simulink model "MSabc_TPM1Base0x2830x291"  (R2023b)
settings: Solver=ode45  StartTime=0.0  StopTime=0.5  MaxStep=h/10  RelTol=1e-3  EnableMultiTasking=on
model workspace (MAT data in the model file):
  J = 0.004
  Lc_v = 0.00255
  R_v = 0.13
  Vmax = 530
  fv = 0.08
  p = 4
  psid0_v = 0.222
values from neighbouring files (symbols this model uses):
  h = 50e-6    (= 5e-05)    [MotorDat_MSTPM1 (1).m]    (also in ParamMinduction0.m; parametres.m = 1e-05)
libraries: simulink x1, spsThreePhaseSineGeneratorLib x1
settings Model: Creator=dgrenier  LastModifiedBy=boris
settings SolverCC: AlgebraicLoopSolver=TrustRegion
settings DataIOCC: LimitDataPoints=on  SaveFormat=Array  SignalLoggingSaveFormat=ModelDataLogs  ReturnWorkspaceOutputs=off
settings OptimizationCC: ExpressionDepthLimit=2147483647  InitFltsAndDblsToZero=on  LifeSpan=inf
settings DebuggingCC: SaveWithParameterizedLinksMsg=none  UnderspecifiedInitializationDetection=Classic  MergeDetectMultiDrivingBlocksExec=none  SignalResolutionControl=TryResolveAllWithWarning  SolverPrmCheckMsg=warning  MultiTaskDSMMsg=warning  MultiTaskCondExecSysMsg=none  FcnCallInpInsideContextMsg=warning  UnconnectedInputMsg=warning  UnconnectedOutputMsg=warning  UnconnectedLineMsg=warning  StateNameClashWarn=warning  SFUnexpectedBacktrackingDiag=warning  SFNoUnconditionalDefaultTransitionDiag=warning  SFExecutionAtInitializationDiag=none  ArithmeticOperatorsInVariantConditions=warning
settings HardwareCC: ProdBitPerPointer=32  ProdBitPerSizeT=32  ProdBitPerPtrDiffT=32  ProdLargestAtomicFloat=None  ProdIntDivRoundTo=Undefined  ProdEndianess=Unspecified  ProdWordSize=32  ProdHWDeviceType=32-bit Generic
settings ModelReferenceCC: EnableRefExpFcnMdlSchedulingChecks=on  PropagateSignalLabelsOutOfModel=off
settings SFSimCC: SimUseLocalCustomCode=off  CustomCodeUndefinedFunction=UseInterfaceOnly
settings RTWCC: RTWUseLocalCustomCode=off  DLArmComputeVersion=19.05
settings CodeAppCC: StateflowObjectComments=on
settings GRTTargetCC: TargetFcnLib=ansi_tfl_tmw.mat  TargetLangStandard=C89/C90 (ANSI)  CombineOutputUpdateFcns=off  GRTInterface=on
settings ConfigComp: CovMetricSettings=dw  CovSaveCumulativeToWorkspaceVar=on  CovSaveSingleToWorkspaceVar=on  CovExternalEMLEnable=off  CovSFcnEnable=off

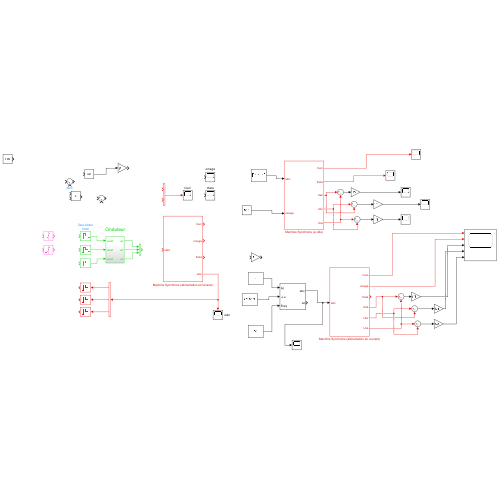
[thumbnail: Simulink's stored preview of the top-level diagram]
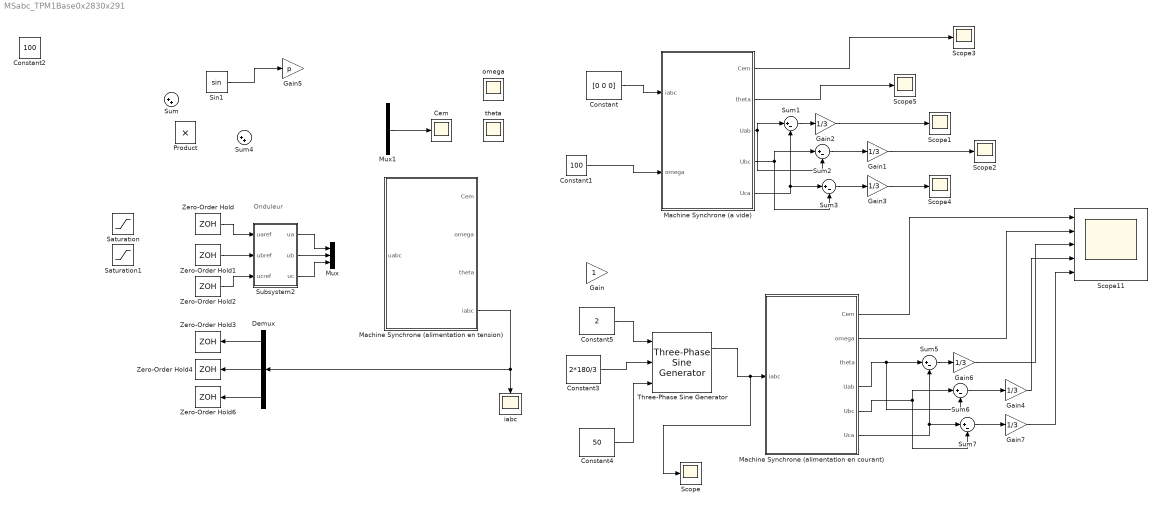
== system MSabc_TPM1Base0x2830x291 ==
  note: Onduleur
  Cem : Scope
  Constant : Constant  Value=[0 0 0]
  Constant1 : Constant  Value=100
  Constant2 : Constant  Value=100
  Constant3 : Constant  Value=2*180/3
  Constant4 : Constant  Value=50
  Constant5 : Constant  Value=2
  Demux : Demux  Outputs=3
  Gain : Gain
  Gain{1..4,6..7} (6 alike) : Gain  Gain=1/3
  Gain5 : Gain  Gain=p
  Machine Synchrone (a vide) : Subsystem
  Machine Synchrone (alimentation en courant) : Subsystem
  Machine Synchrone (alimentation en tension) : Subsystem
  Mux : Mux  Inputs=3
  Mux1 : Mux  Inputs=2
  Product : Product
  Saturation : Saturate  UpperLimit=Vmax/2  LowerLimit=-Vmax/2
  Saturation1 : Saturate  UpperLimit=Vmax/2  LowerLimit=-Vmax/2
  Scope{,1..5} (6 alike) : Scope
  Scope11 : Scope  NumInputPorts=5
  Sin1 : Trigonometry
  Subsystem2 : Subsystem
  Sum : Sum  Inputs=|++
  Sum{1..3,5..7} (6 alike) : Sum  Inputs=|+-
  Sum4 : Sum  Inputs=|++
  Three-Phase Sine Generator : spsThreePhaseSineGeneratorLib/Three-Phase Sine Generator  Ts=0
      settings: LibrarySourceBlock=|
      | sps_lib/Sources/Signal Generator Sources/Three-Phase
      | Sine Generator
  Zero-Order Hold{,1..4,6} (6 alike) : ZeroOrderHold  SampleTime=h
  iabc : Scope
  omega : Scope
  theta : Scope
  wires:
  Subsystem2/1(ua) -> Mux/1
  Subsystem2/2(ub) -> Mux/2
  Subsystem2/3(uc) -> Mux/3
  Mux1/1 -> Cem/1
  Zero-Order Hold/1 -> Subsystem2/1(uaref)
  Zero-Order Hold1/1 -> Subsystem2/2(ubref)
  Zero-Order Hold2/1 -> Subsystem2/3(ucref)
  Demux/1 -> Zero-Order Hold3/1
  Demux/2 -> Zero-Order Hold4/1
  Demux/3 -> Zero-Order Hold6/1
  Machine Synchrone (alimentation en tension)/4(iabc) -> Demux/1, iabc/1
  Constant/1 -> Machine Synchrone (a vide)/1(iabc)
  Constant1/1 -> Machine Synchrone (a vide)/2(omega)
  Sin1/1 -> Gain5/1
  Machine Synchrone (a vide)/3(Uab) -> Sum1/1, Sum2/2
  Machine Synchrone (a vide)/5(Uca) -> Sum3/1, Sum1/2
  Sum1/1 -> Gain2/1
  Gain2/1 -> Scope1/1
  Sum2/1 -> Gain1/1
  Machine Synchrone (a vide)/4(Ubc) -> Sum2/1, Sum3/2
  Gain1/1 -> Scope2/1
  Sum3/1 -> Gain3/1
  Gain3/1 -> Scope4/1
  Machine Synchrone (a vide)/1(Cem) -> Scope3/1
  Machine Synchrone (a vide)/2(theta) -> Scope5/1
  Three-Phase Sine Generator/1 -> Scope/1, Machine Synchrone (alimentation en courant)/1(iabc)
  Constant3/1 -> Three-Phase Sine Generator/2
  Sum6/1 -> Gain4/1
  Sum7/1 -> Gain7/1
  Sum5/1 -> Gain6/1
  Machine Synchrone (alimentation en courant)/5(Ubc) -> Sum6/1, Sum7/2
  Machine Synchrone (alimentation en courant)/6(Uca) -> Sum7/1, Sum5/2
  Gain4/1 -> Scope11/4
  Gain6/1 -> Scope11/3
  Gain7/1 -> Scope11/5
  Machine Synchrone (alimentation en courant)/4(Uab) -> Sum5/1, Sum6/2
  Machine Synchrone (alimentation en courant)/1(Cem) -> Scope11/1
  Machine Synchrone (alimentation en courant)/2(omega) -> Scope11/2
  Constant4/1 -> Three-Phase Sine Generator/3
  Constant5/1 -> Three-Phase Sine Generator/1

== system MSabc_TPM1Base0x2830x291/Machine Synchrone (a vide) ==
  iabc : Inport
  omega : Inport  Port=2
  Integrator1 : Integrator  InitialCondition=pi/6  WrapState=on
  Machine Synchrone1 : Subsystem
  Sum : Sum  Inputs=|+-
  Sum1 : Sum  Inputs=|+-
  Sum2 : Sum  Inputs=-+|
  Cem : Outport
  theta : Outport  Port=2
  Uab : Outport  Port=3
  Ubc : Outport  Port=4
  Uca : Outport  Port=5
  wires:
  iabc/1 -> Machine Synchrone1/3(iabc)
  Integrator1/1 -> Machine Synchrone1/2(thetam), theta/1
  Machine Synchrone1/1(Cem) -> Cem/1
  omega/1 -> Machine Synchrone1/1(omegam), Integrator1/1
  Machine Synchrone1/2(ua) -> Sum2/1, Sum/1
  Machine Synchrone1/3(ub) -> Sum/2, Sum1/1
  Sum1/1 -> Ubc/1
  Sum/1 -> Uab/1
  Machine Synchrone1/4(uc) -> Sum1/2, Sum2/2
  Sum2/1 -> Uca/1

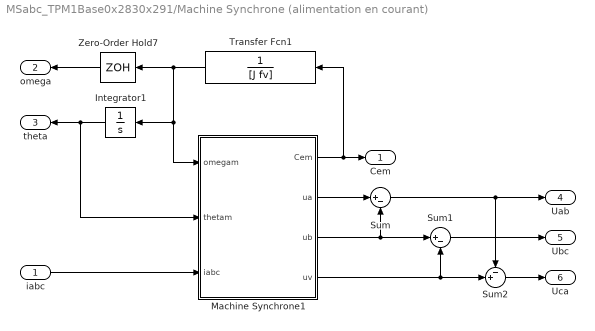
== system MSabc_TPM1Base0x2830x291/Machine Synchrone (alimentation en courant) ==
  iabc : Inport
  Integrator1 : Integrator  InitialCondition=pi/6  WrapState=on
  Machine Synchrone1 : Subsystem
  Sum : Sum  Inputs=|+-
  Sum1 : Sum  Inputs=|+-
  Sum2 : Sum  Inputs=-+|
  Transfer Fcn1 : TransferFcn  Denominator=[J fv]
  Zero-Order Hold7 : ZeroOrderHold  SampleTime=h
  Cem : Outport
  omega : Outport  Port=2
  theta : Outport  Port=3
  Uab : Outport  Port=4
  Ubc : Outport  Port=5
  Uca : Outport  Port=6
  wires:
  iabc/1 -> Machine Synchrone1/3(iabc)
  Integrator1/1 -> Machine Synchrone1/2(thetam), theta/1
  Transfer Fcn1/1 -> Machine Synchrone1/1(omegam), Integrator1/1, Zero-Order Hold7/1
  Zero-Order Hold7/1 -> omega/1
  Machine Synchrone1/1(Cem) -> Cem/1, Transfer Fcn1/1
  Sum/1 -> Sum2/1, Uab/1
  Machine Synchrone1/4(uv) -> Sum2/2, Sum1/2
  Machine Synchrone1/3(ub) -> Sum/2, Sum1/1
  Sum1/1 -> Ubc/1
  Sum2/1 -> Uca/1
  Machine Synchrone1/2(ua) -> Sum/1

== system MSabc_TPM1Base0x2830x291/Machine Synchrone (alimentation en tension) ==
  uabc : Inport
  Integrator : Integrator  InitialCondition=pi/6  WrapState=on
  Machine Synchrone : Subsystem
  Transfer Fcn4 : TransferFcn  Denominator=[J fv]
  Zero-Order Hold5 : ZeroOrderHold  SampleTime=h
  Cem : Outport
  omega : Outport  Port=2
  theta : Outport  Port=3
  iabc : Outport  Port=4
  wires:
  Zero-Order Hold5/1 -> omega/1
  Machine Synchrone/2(iabc) -> iabc/1
  Integrator/1 -> Machine Synchrone/2(thetam), theta/1
  uabc/1 -> Machine Synchrone/3(uabc)
  Machine Synchrone/1(Cem) -> Cem/1, Transfer Fcn4/1
  Transfer Fcn4/1 -> Machine Synchrone/1(omegam), Integrator/1, Zero-Order Hold5/1

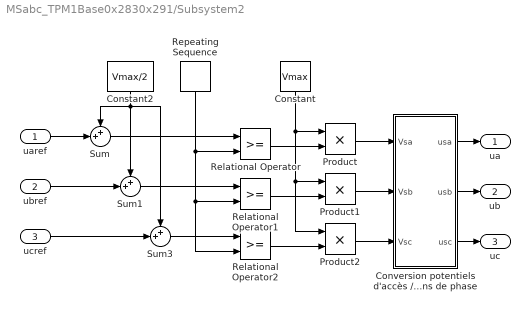
== system MSabc_TPM1Base0x2830x291/Subsystem2 ==
  uaref : Inport
  ubref : Inport  Port=2
  ucref : Inport  Port=3
  Constant : Constant  Value=Vmax
  Constant2 : Constant  Value=Vmax/2
  Conversion potentiels d'accès / tensions de phase : Subsystem
  Product : Product  RndMeth=Zero
  Product1 : Product  RndMeth=Zero
  Product2 : Product  RndMeth=Zero
  Relational Operator : RelationalOperator  OutDataTypeStr=boolean  ZeroCross=off  InputSameDT=off
  Relational Operator1 : RelationalOperator  OutDataTypeStr=boolean  ZeroCross=off  InputSameDT=off
  Relational Operator2 : RelationalOperator  OutDataTypeStr=boolean  ZeroCross=off  InputSameDT=off
  Repeating Sequence : simulink/Sources/Repeating Sequence  rep_seq_t=[0 h 2*h]  rep_seq_y=[0 Vmax 0]
  Sum : Sum  Inputs=++|
  Sum1 : Sum  Inputs=++|
  Sum3 : Sum  Inputs=++|
  ua : Outport
  ub : Outport  Port=2
  uc : Outport  Port=3
  wires:
  Constant2/1 -> Sum3/1, Sum/1, Sum1/1
  Product2/1 -> Conversion potentiels d'accès / tensions de phase/3(Vsc)
  Product1/1 -> Conversion potentiels d'accès / tensions de phase/2(Vsb)
  Product/1 -> Conversion potentiels d'accès / tensions de phase/1(Vsa)
  Relational Operator2/1 -> Product2/2
  Sum3/1 -> Relational Operator2/1
  Sum1/1 -> Relational Operator1/1
  Sum/1 -> Relational Operator/1
  Relational Operator1/1 -> Product1/2
  Constant/1 -> Product2/1, Product1/1, Product/1
  Relational Operator/1 -> Product/2
  Repeating Sequence/1 -> Relational Operator2/2, Relational Operator1/2, Relational Operator/2
  Conversion potentiels d'accès / tensions de phase/3(usc) -> uc/1
  Conversion potentiels d'accès / tensions de phase/2(usb) -> ub/1
  Conversion potentiels d'accès / tensions de phase/1(usa) -> ua/1
  ucref/1 -> Sum3/2
  uaref/1 -> Sum/2
  ubref/1 -> Sum1/2

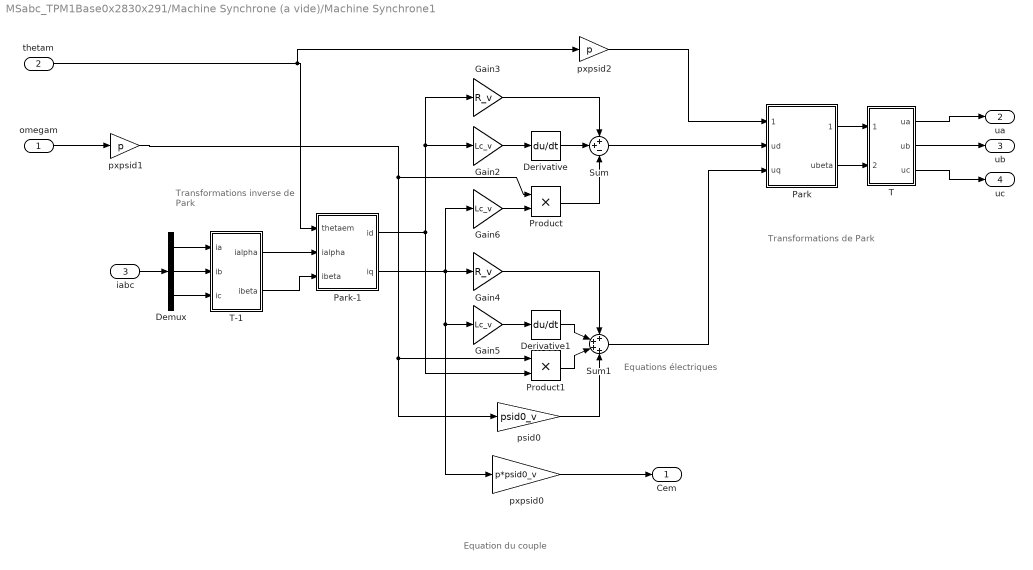
== system MSabc_TPM1Base0x2830x291/Machine Synchrone (a vide)/Machine Synchrone1 ==
  note: Transformations de Park
  note: Transformations
      | inverse de Park
  note: Equation du couple
  note: Equations électriques
  omegam : Inport
  thetam : Inport  Port=2
  iabc : Inport  Port=3
  Demux : Demux  Outputs=3
  Derivative : Derivative
  Derivative1 : Derivative
  Gain2 : Gain  Gain=Lc_v
  Gain3 : Gain  Gain=R_v
  Gain4 : Gain  Gain=R_v
  Gain5 : Gain  Gain=Lc_v
  Gain6 : Gain  Gain=Lc_v
  Park : Subsystem
  Park-1 : Subsystem
  Product : Product  RndMeth=Zero
  Product1 : Product  RndMeth=Zero
  Sum : Sum  Inputs=++-
  Sum1 : Sum  Inputs=++++
  T : Subsystem
  T-1 : Subsystem
  psid0 : Gain  Gain=psid0_v
  pxpsid0 : Gain  Gain=p*psid0_v
  pxpsid1 : Gain  Gain=p
  pxpsid2 : Gain  Gain=p
  Cem : Outport
  ua : Outport  Port=2
  ub : Outport  Port=3
  uc : Outport  Port=4
  wires:
  pxpsid0/1 -> Cem/1
  T/3(uc) -> uc/1
  T/2(ub) -> ub/1
  Demux/3 -> T-1/3(ic)
  Demux/2 -> T-1/2(ib)
  Park/1(ualpha) -> T/1(ialpha)
  Park/2(ubeta) -> T/2(ibeta)
  Sum/1 -> Park/2(ud)
  pxpsid1/1 -> psid0/1, Product1/1, Product/1
  T-1/2(ibeta) -> Park-1/3(ibeta)
  T-1/1(ialpha) -> Park-1/2(ialpha)
  T/1(ua) -> ua/1
  iabc/1 -> Demux/1
  Demux/1 -> T-1/1(ia)
  omegam/1 -> pxpsid1/1
  thetam/1 -> pxpsid2/1, Park-1/1(thetaem)
  Park-1/1(id) -> Product1/2, Gain3/1, Gain2/1
  Gain2/1 -> Derivative/1
  Gain3/1 -> Sum/1
  Derivative/1 -> Sum/2
  Product/1 -> Sum/3
  Gain6/1 -> Product/2
  Park-1/2(iq) -> Gain5/1, pxpsid0/1, Gain4/1, Gain6/1
  Gain5/1 -> Derivative1/1
  Derivative1/1 -> Sum1/2
  Gain4/1 -> Sum1/1
  Product1/1 -> Sum1/3
  psid0/1 -> Sum1/4
  Sum1/1 -> Park/3(uq)
  pxpsid2/1 -> Park/1(thetaem)

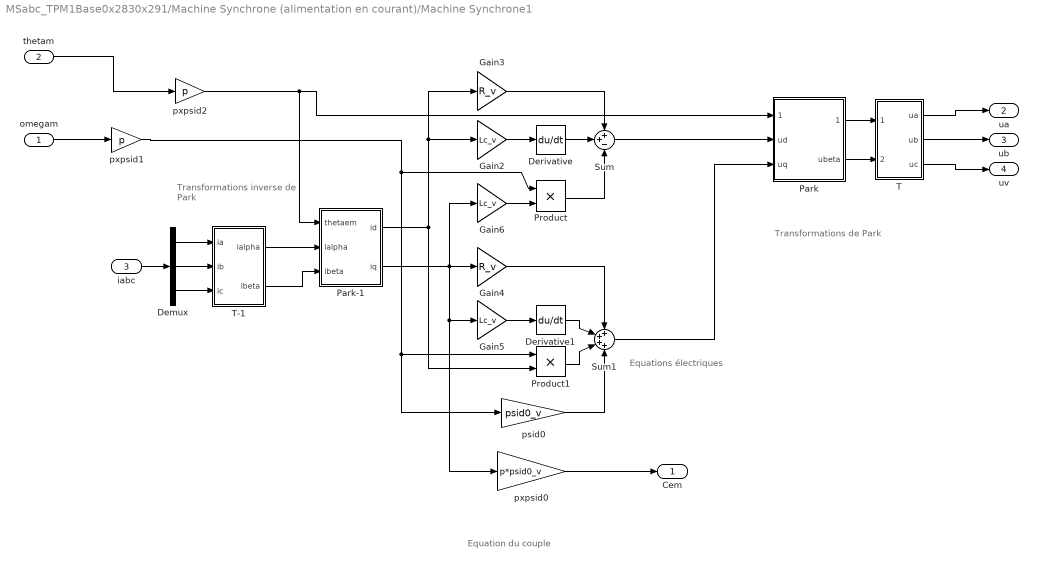
== system MSabc_TPM1Base0x2830x291/Machine Synchrone (alimentation en courant)/Machine Synchrone1 ==
  note: Transformations de Park
  note: Transformations
      | inverse de Park
  note: Equation du couple
  note: Equations électriques
  omegam : Inport
  thetam : Inport  Port=2
  iabc : Inport  Port=3
  Demux : Demux  Outputs=3
  Derivative : Derivative
  Derivative1 : Derivative
  Gain2 : Gain  Gain=Lc_v
  Gain3 : Gain  Gain=R_v
  Gain4 : Gain  Gain=R_v
  Gain5 : Gain  Gain=Lc_v
  Gain6 : Gain  Gain=Lc_v
  Park : Subsystem
  Park-1 : Subsystem
  Product : Product  RndMeth=Zero
  Product1 : Product  RndMeth=Zero
  Sum : Sum  Inputs=++-
  Sum1 : Sum  Inputs=++++
  T : Subsystem
  T-1 : Subsystem
  psid0 : Gain  Gain=psid0_v
  pxpsid0 : Gain  Gain=p*psid0_v
  pxpsid1 : Gain  Gain=p
  pxpsid2 : Gain  Gain=p
  Cem : Outport
  ua : Outport  Port=2
  ub : Outport  Port=3
  uv : Outport  Port=4
  wires:
  pxpsid0/1 -> Cem/1
  T/2(ub) -> ub/1
  Demux/3 -> T-1/3(ic)
  Demux/2 -> T-1/2(ib)
  Park/1(ualpha) -> T/1(ialpha)
  Park/2(ubeta) -> T/2(ibeta)
  Sum/1 -> Park/2(ud)
  pxpsid1/1 -> psid0/1, Product1/1, Product/1
  T-1/2(ibeta) -> Park-1/3(ibeta)
  T-1/1(ialpha) -> Park-1/2(ialpha)
  T/1(ua) -> ua/1
  iabc/1 -> Demux/1
  Demux/1 -> T-1/1(ia)
  omegam/1 -> pxpsid1/1
  Park-1/1(id) -> Product1/2, Gain3/1, Gain2/1
  Gain2/1 -> Derivative/1
  Gain3/1 -> Sum/1
  Derivative/1 -> Sum/2
  Product/1 -> Sum/3
  Gain6/1 -> Product/2
  Park-1/2(iq) -> Gain5/1, pxpsid0/1, Gain4/1, Gain6/1
  Gain5/1 -> Derivative1/1
  Derivative1/1 -> Sum1/2
  Gain4/1 -> Sum1/1
  Product1/1 -> Sum1/3
  psid0/1 -> Sum1/4
  Sum1/1 -> Park/3(uq)
  T/3(uc) -> uv/1
  pxpsid2/1 -> Park-1/1(thetaem), Park/1(thetaem)
  thetam/1 -> pxpsid2/1

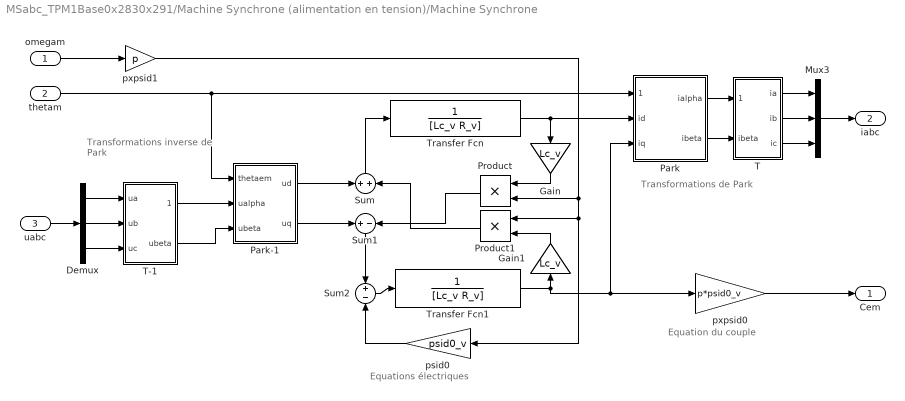
== system MSabc_TPM1Base0x2830x291/Machine Synchrone (alimentation en tension)/Machine Synchrone ==
  note: Transformations de Park
  note: Transformations
      | inverse de Park
  note: Equation du couple
  note: Equations électriques
  omegam : Inport
  thetam : Inport  Port=2
  uabc : Inport  Port=3
  Demux : Demux  Outputs=3
  Gain : Gain  Gain=Lc_v
  Gain1 : Gain  Gain=Lc_v
  Mux3 : Mux  Inputs=3
  Park : Subsystem
  Park-1 : Subsystem
  Product : Product  RndMeth=Zero
  Product1 : Product  RndMeth=Zero
  Sum : Sum  Inputs=+|+
  Sum1 : Sum  Inputs=+|-
  Sum2 : Sum  Inputs=+|-
  T : Subsystem
  T-1 : Subsystem
  Transfer Fcn : TransferFcn  Denominator=[Lc_v R_v]
  Transfer Fcn1 : TransferFcn  Denominator=[Lc_v R_v]
  psid0 : Gain  Gain=psid0_v
  pxpsid0 : Gain  Gain=p*psid0_v
  pxpsid1 : Gain  Gain=p
  Cem : Outport
  iabc : Outport  Port=2
  wires:
  pxpsid0/1 -> Cem/1
  T/3(ic) -> Mux3/3
  T/2(ib) -> Mux3/2
  Demux/3 -> T-1/3(uc)
  Demux/2 -> T-1/2(ub)
  Park/1(ialpha) -> T/1(ialpha)
  Park/2(ibeta) -> T/2(ibeta)
  psid0/1 -> Sum2/2
  Gain1/1 -> Product1/2
  Transfer Fcn1/1 -> pxpsid0/1, Park/3(iq), Gain1/1
  Sum2/1 -> Transfer Fcn1/1
  Sum1/1 -> Sum2/1
  Sum/1 -> Transfer Fcn/1
  Product1/1 -> Sum/2
  Product/1 -> Sum1/2
  Transfer Fcn/1 -> Gain/1, Park/2(id)
  Gain/1 -> Product/1
  Park-1/2(uq) -> Sum1/1
  Park-1/1(ud) -> Sum/1
  T-1/2(ubeta) -> Park-1/3(ubeta)
  T-1/1(ualpha) -> Park-1/2(ualpha)
  T/1(ia) -> Mux3/1
  Mux3/1 -> iabc/1
  uabc/1 -> Demux/1
  Demux/1 -> T-1/1(ua)
  omegam/1 -> pxpsid1/1
  pxpsid1/1 -> Product/2, Product1/1, psid0/1
  thetam/1 -> Park/1(thetaem), Park-1/1(thetaem)

== system MSabc_TPM1Base0x2830x291/Subsystem2/Conversion potentiels d'accès // tensions de phase ==
  Vsa : Inport
  Vsb : Inport  Port=2
  Vsc : Inport  Port=3
  Gain : Gain  Gain=1/3
  Sum : Sum  Inputs=+++
  Sum1 : Sum  Inputs=-+|
  Sum2 : Sum  Inputs=-+|
  Sum3 : Sum  Inputs=-+|
  usa : Outport
  usb : Outport  Port=2
  usc : Outport  Port=3
  wires:
  Sum3/1 -> usc/1
  Sum2/1 -> usb/1
  Sum1/1 -> usa/1
  Gain/1 -> Sum3/1, Sum2/1, Sum1/1
  Sum/1 -> Gain/1
  Vsc/1 -> Sum/3, Sum3/2
  Vsb/1 -> Sum/2, Sum2/2
  Vsa/1 -> Sum/1, Sum1/2

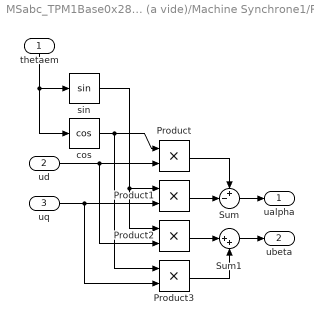
== system MSabc_TPM1Base0x2830x291/Machine Synchrone (a vide)/Machine Synchrone1/Park ==
  thetaem : Inport
  ud : Inport  Port=2
  uq : Inport  Port=3
  Product{,1..3} (4 alike) : Product  RndMeth=Zero
  Sum : Sum  Inputs=+-|
  Sum1 : Sum  Inputs=|++
  cos : Trigonometry  Operator=cos
  sin : Trigonometry
  ualpha : Outport
  ubeta : Outport  Port=2
  wires:
  Sum1/1 -> ubeta/1
  Sum/1 -> ualpha/1
  uq/1 -> Product3/2, Product1/2
  ud/1 -> Product2/2, Product/2
  Product3/1 -> Sum1/2
  Product2/1 -> Sum1/1
  Product1/1 -> Sum/2
  Product/1 -> Sum/1
  sin/1 -> Product2/1, Product1/1
  cos/1 -> Product3/1, Product/1
  thetaem/1 -> sin/1, cos/1

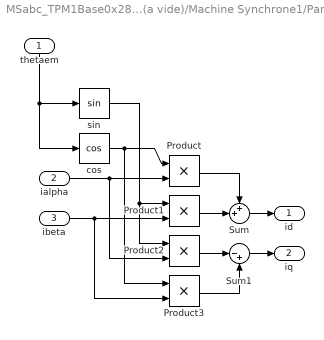
== system MSabc_TPM1Base0x2830x291/Machine Synchrone (a vide)/Machine Synchrone1/Park-1 ==
  thetaem : Inport
  ialpha : Inport  Port=2
  ibeta : Inport  Port=3
  Product{,1..3} (4 alike) : Product  RndMeth=Zero
  Sum : Sum  Inputs=++|
  Sum1 : Sum  Inputs=|-+
  cos : Trigonometry  Operator=cos
  sin : Trigonometry
  id : Outport
  iq : Outport  Port=2
  wires:
  Sum1/1 -> iq/1
  Sum/1 -> id/1
  ibeta/1 -> Product3/2, Product1/2
  ialpha/1 -> Product2/2, Product/2
  Product3/1 -> Sum1/2
  Product2/1 -> Sum1/1
  Product1/1 -> Sum/2
  Product/1 -> Sum/1
  sin/1 -> Product2/1, Product1/1
  cos/1 -> Product3/1, Product/1
  thetaem/1 -> sin/1, cos/1

== system MSabc_TPM1Base0x2830x291/Machine Synchrone (a vide)/Machine Synchrone1/T ==
  ialpha : Inport
  ibeta : Inport  Port=2
  1/sqrt(6) : Gain  Gain=1/sqrt(6)
  Sum4 : Sum  Inputs=|--
  Sum5 : Sum  Inputs=|-+
  sqrt(2)/2 : Gain  Gain=sqrt(2)/2
  sqrt(2/3) : Gain  Gain=sqrt(2/3)
  ua : Outport
  ub : Outport  Port=2
  uc : Outport  Port=3
  wires:
  ibeta/1 -> sqrt(2)/2/1
  Sum4/1 -> uc/1
  Sum5/1 -> ub/1
  sqrt(2/3)/1 -> ua/1
  sqrt(2)/2/1 -> Sum4/2, Sum5/2
  1/sqrt(6)/1 -> Sum4/1, Sum5/1
  ialpha/1 -> 1/sqrt(6)/1, sqrt(2/3)/1

== system MSabc_TPM1Base0x2830x291/Machine Synchrone (a vide)/Machine Synchrone1/T-1 ==
  ia : Inport
  ib : Inport  Port=2
  ic : Inport  Port=3
  -1/2 : Gain  Gain=-0.5
  Sum : Sum  Inputs=|++
  Sum1 : Sum  Inputs=|++
  Sum2 : Sum  Inputs=+-|
  sqrt(2)/2 : Gain  Gain=sqrt(2)/2
  sqrt(2/3) : Gain  Gain=sqrt(2/3)
  ialpha : Outport
  ibeta : Outport  Port=2
  wires:
  sqrt(2)/2/1 -> ibeta/1
  sqrt(2/3)/1 -> ialpha/1
  ia/1 -> Sum1/1
  Sum2/1 -> sqrt(2)/2/1
  Sum1/1 -> sqrt(2/3)/1
  -1/2/1 -> Sum1/2
  Sum/1 -> -1/2/1
  ic/1 -> Sum2/2, Sum/2
  ib/1 -> Sum2/1, Sum/1

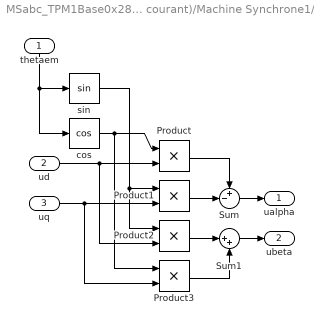
== system MSabc_TPM1Base0x2830x291/Machine Synchrone (alimentation en courant)/Machine Synchrone1/Park ==
  thetaem : Inport
  ud : Inport  Port=2
  uq : Inport  Port=3
  Product{,1..3} (4 alike) : Product  RndMeth=Zero
  Sum : Sum  Inputs=+-|
  Sum1 : Sum  Inputs=|++
  cos : Trigonometry  Operator=cos
  sin : Trigonometry
  ualpha : Outport
  ubeta : Outport  Port=2
  wires:
  Sum1/1 -> ubeta/1
  Sum/1 -> ualpha/1
  uq/1 -> Product3/2, Product1/2
  ud/1 -> Product2/2, Product/2
  Product3/1 -> Sum1/2
  Product2/1 -> Sum1/1
  Product1/1 -> Sum/2
  Product/1 -> Sum/1
  sin/1 -> Product2/1, Product1/1
  cos/1 -> Product3/1, Product/1
  thetaem/1 -> sin/1, cos/1

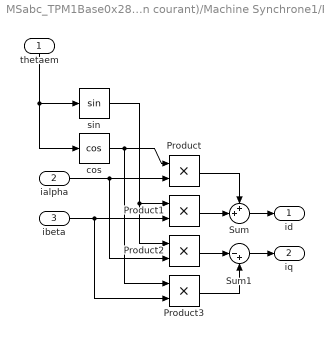
== system MSabc_TPM1Base0x2830x291/Machine Synchrone (alimentation en courant)/Machine Synchrone1/Park-1 ==
  thetaem : Inport
  ialpha : Inport  Port=2
  ibeta : Inport  Port=3
  Product{,1..3} (4 alike) : Product  RndMeth=Zero
  Sum : Sum  Inputs=++|
  Sum1 : Sum  Inputs=|-+
  cos : Trigonometry  Operator=cos
  sin : Trigonometry
  id : Outport
  iq : Outport  Port=2
  wires:
  Sum1/1 -> iq/1
  Sum/1 -> id/1
  ibeta/1 -> Product3/2, Product1/2
  ialpha/1 -> Product2/2, Product/2
  Product3/1 -> Sum1/2
  Product2/1 -> Sum1/1
  Product1/1 -> Sum/2
  Product/1 -> Sum/1
  sin/1 -> Product2/1, Product1/1
  cos/1 -> Product3/1, Product/1
  thetaem/1 -> sin/1, cos/1

== system MSabc_TPM1Base0x2830x291/Machine Synchrone (alimentation en courant)/Machine Synchrone1/T ==
  ialpha : Inport
  ibeta : Inport  Port=2
  1/sqrt(6) : Gain  Gain=1/sqrt(6)
  Sum4 : Sum  Inputs=|--
  Sum5 : Sum  Inputs=|-+
  sqrt(2)/2 : Gain  Gain=sqrt(2)/2
  sqrt(2/3) : Gain  Gain=sqrt(2/3)
  ua : Outport
  ub : Outport  Port=2
  uc : Outport  Port=3
  wires:
  ibeta/1 -> sqrt(2)/2/1
  Sum4/1 -> uc/1
  Sum5/1 -> ub/1
  sqrt(2/3)/1 -> ua/1
  sqrt(2)/2/1 -> Sum4/2, Sum5/2
  1/sqrt(6)/1 -> Sum4/1, Sum5/1
  ialpha/1 -> 1/sqrt(6)/1, sqrt(2/3)/1

== system MSabc_TPM1Base0x2830x291/Machine Synchrone (alimentation en courant)/Machine Synchrone1/T-1 ==
  ia : Inport
  ib : Inport  Port=2
  ic : Inport  Port=3
  -1/2 : Gain  Gain=-0.5
  Sum : Sum  Inputs=|++
  Sum1 : Sum  Inputs=|++
  Sum2 : Sum  Inputs=+-|
  sqrt(2)/2 : Gain  Gain=sqrt(2)/2
  sqrt(2/3) : Gain  Gain=sqrt(2/3)
  ialpha : Outport
  ibeta : Outport  Port=2
  wires:
  sqrt(2)/2/1 -> ibeta/1
  sqrt(2/3)/1 -> ialpha/1
  ia/1 -> Sum1/1
  Sum2/1 -> sqrt(2)/2/1
  Sum1/1 -> sqrt(2/3)/1
  -1/2/1 -> Sum1/2
  Sum/1 -> -1/2/1
  ic/1 -> Sum2/2, Sum/2
  ib/1 -> Sum2/1, Sum/1

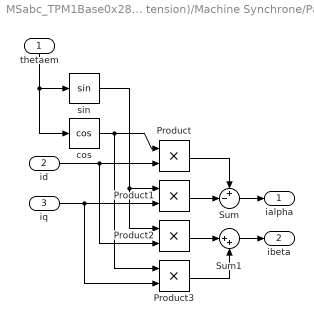
== system MSabc_TPM1Base0x2830x291/Machine Synchrone (alimentation en tension)/Machine Synchrone/Park ==
  thetaem : Inport
  id : Inport  Port=2
  iq : Inport  Port=3
  Product{,1..3} (4 alike) : Product  RndMeth=Zero
  Sum : Sum  Inputs=+-|
  Sum1 : Sum  Inputs=|++
  cos : Trigonometry  Operator=cos
  sin : Trigonometry
  ialpha : Outport
  ibeta : Outport  Port=2
  wires:
  Sum1/1 -> ibeta/1
  Sum/1 -> ialpha/1
  iq/1 -> Product3/2, Product1/2
  id/1 -> Product2/2, Product/2
  Product3/1 -> Sum1/2
  Product2/1 -> Sum1/1
  Product1/1 -> Sum/2
  Product/1 -> Sum/1
  sin/1 -> Product2/1, Product1/1
  cos/1 -> Product3/1, Product/1
  thetaem/1 -> sin/1, cos/1

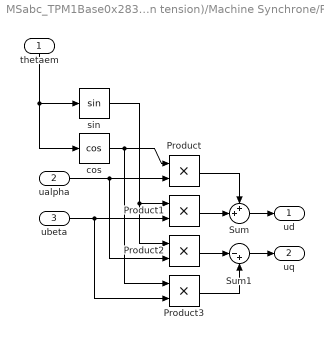
== system MSabc_TPM1Base0x2830x291/Machine Synchrone (alimentation en tension)/Machine Synchrone/Park-1 ==
  thetaem : Inport
  ualpha : Inport  Port=2
  ubeta : Inport  Port=3
  Product{,1..3} (4 alike) : Product  RndMeth=Zero
  Sum : Sum  Inputs=++|
  Sum1 : Sum  Inputs=|-+
  cos : Trigonometry  Operator=cos
  sin : Trigonometry
  ud : Outport
  uq : Outport  Port=2
  wires:
  Sum1/1 -> uq/1
  Sum/1 -> ud/1
  ubeta/1 -> Product3/2, Product1/2
  ualpha/1 -> Product2/2, Product/2
  Product3/1 -> Sum1/2
  Product2/1 -> Sum1/1
  Product1/1 -> Sum/2
  Product/1 -> Sum/1
  sin/1 -> Product2/1, Product1/1
  cos/1 -> Product3/1, Product/1
  thetaem/1 -> sin/1, cos/1

== system MSabc_TPM1Base0x2830x291/Machine Synchrone (alimentation en tension)/Machine Synchrone/T ==
  ialpha : Inport
  ibeta : Inport  Port=2
  1/sqrt(6) : Gain  Gain=1/sqrt(6)
  Sum4 : Sum  Inputs=|--
  Sum5 : Sum  Inputs=|-+
  sqrt(2)/2 : Gain  Gain=sqrt(2)/2
  sqrt(2/3) : Gain  Gain=sqrt(2/3)
  ia : Outport
  ib : Outport  Port=2
  ic : Outport  Port=3
  wires:
  ibeta/1 -> sqrt(2)/2/1
  Sum4/1 -> ic/1
  Sum5/1 -> ib/1
  sqrt(2/3)/1 -> ia/1
  sqrt(2)/2/1 -> Sum4/2, Sum5/2
  1/sqrt(6)/1 -> Sum4/1, Sum5/1
  ialpha/1 -> 1/sqrt(6)/1, sqrt(2/3)/1

== system MSabc_TPM1Base0x2830x291/Machine Synchrone (alimentation en tension)/Machine Synchrone/T-1 ==
  ua : Inport
  ub : Inport  Port=2
  uc : Inport  Port=3
  -1/2 : Gain  Gain=-0.5
  Sum : Sum  Inputs=|++
  Sum1 : Sum  Inputs=|++
  Sum2 : Sum  Inputs=+-|
  sqrt(2)/2 : Gain  Gain=sqrt(2)/2
  sqrt(2/3) : Gain  Gain=sqrt(2/3)
  ualpha : Outport
  ubeta : Outport  Port=2
  wires:
  sqrt(2)/2/1 -> ubeta/1
  sqrt(2/3)/1 -> ualpha/1
  ua/1 -> Sum1/1
  Sum2/1 -> sqrt(2)/2/1
  Sum1/1 -> sqrt(2/3)/1
  -1/2/1 -> Sum1/2
  Sum/1 -> -1/2/1
  uc/1 -> Sum2/2, Sum/2
  ub/1 -> Sum2/1, Sum/1
